simulink model "VCUInterfaceHandler"  (R2024a)
settings: Solver=VariableStepAuto  StartTime=0.0  StopTime=10.0  RelTol=1e-3
libraries: simulink x1
settings Model: DataDictionary=BMS_System_Arch_dict.sldd  Creator=ghourabi  LastModifiedBy=ghourabi

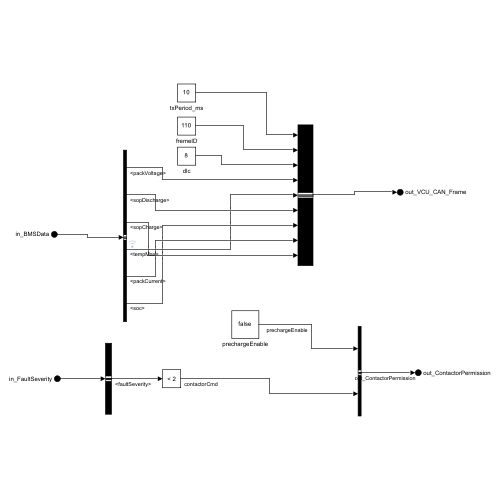
[thumbnail: Simulink's stored preview of the top-level diagram]
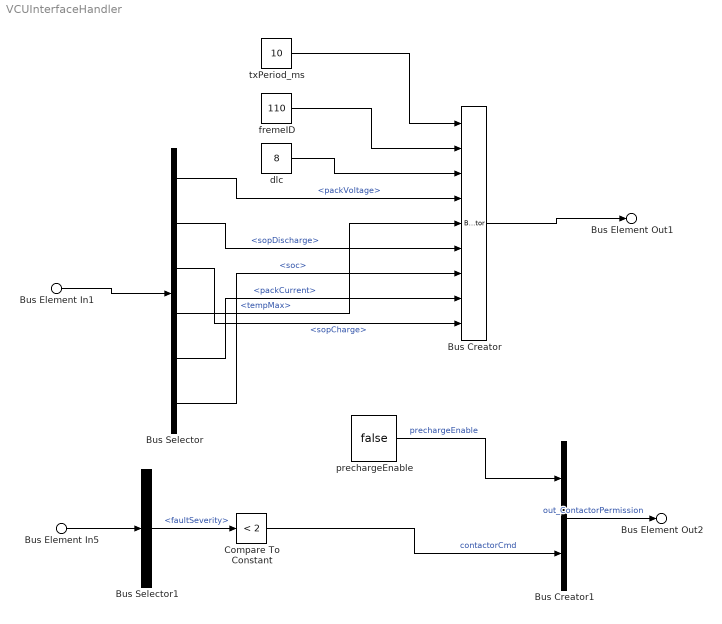
== system VCUInterfaceHandler ==
  Bus Element In1 : Inport  PortName=in_BMSData
  Bus Element In5 : Inport  Port=2  PortName=in_FaultSeverity
  Bus Creator : BusCreator  Inputs=9
  Bus Creator1 : BusCreator  Inputs=2
  Bus Selector : BusSelector  OutputSignals=packVoltage,sopDischarge,sopCharge,tempMax,packCurrent,soc
  Bus Selector1 : BusSelector  OutputSignals=faultSeverity
  Compare To Constant : simulink/Logic and Bit Operations/Compare To Constant  relop=<  const=2  OutDataTypeStr=uint8
  dlc : Constant  Value=8
  fremeID : Constant  Value=110
  prechargeEnable : Constant  Value=false
  txPeriod_ms : Constant  Value=10
  Bus Element Out1 : Outport  PortName=out_VCU_CAN_Frame
  Bus Element Out2 : Outport  Port=2  PortName=out_ContactorPermission
  wires:
  dlc/1 -> Bus Creator/3
  Bus Selector/1 -> Bus Creator/4  "<packVoltage>"
  fremeID/1 -> Bus Creator/2
  Bus Creator/1 -> Bus Element Out1/1
  txPeriod_ms/1 -> Bus Creator/1
  Bus Element In1/1 -> Bus Selector/1
  Bus Element In5/1 -> Bus Selector1/1
  Bus Selector1/1 -> Compare To Constant/1  "<faultSeverity>"
  Compare To Constant/1 -> Bus Creator1/2  "contactorCmd"
  prechargeEnable/1 -> Bus Creator1/1  "prechargeEnable"
  Bus Creator1/1 -> Bus Element Out2/1  "out_ContactorPermission"
  Bus Selector/2 -> Bus Creator/6  "<sopDischarge>"
  Bus Selector/3 -> Bus Creator/9  "<sopCharge>"
  Bus Selector/5 -> Bus Creator/8  "<packCurrent>"
  Bus Selector/6 -> Bus Creator/7  "<soc>"
  Bus Selector/4 -> Bus Creator/5  "<tempMax>"
